simulink model "PARED_SIM_SFR"  (R2018a)
settings: Solver=ode45  StartTime=0.0  StopTime=30  RelTol=1e-6  AbsTol=1e-9  EnableMultiTasking=on
values from neighbouring files (symbols this model uses):
  d0 = 100    [CONTROL_SEGWAY.m]
  matAp = [-1/Tm_w 0 0 ; 1 0 0 ; 1000*xA 1000*va0 0]    [CONTROL_SEGWAY.m]
  matBp = [ Km_w/Tm_w 0 0; 0 -1 0; 0 0 0]    [CONTROL_SEGWAY.m]
  matCp = eye(3)    [CONTROL_SEGWAY.m]
  matDp = zeros(3,3)    [CONTROL_SEGWAY.m]
  param_pared = [Km_w Tm_w xA yA]    [CONTROL_SEGWAY.m]
  ts = 5e-3    (= 0.005)    [CONTROL_SEGWAY.m]
  va0 = 0.15    [CONTROL_SEGWAY.m]
undefined symbols (not defined in the file or in its folder): Kcd_pared
settings Model: Creator=zamora  LastModifiedBy=zamora
settings SolverCC: AutoScaleAbsTol=off
settings DataIOCC: LimitDataPoints=on  SaveFormat=Array  SignalLoggingSaveFormat=ModelDataLogs
settings OptimizationCC: ExpressionDepthLimit=2147483647  LifeSpan=inf
settings DebuggingCC: UnderspecifiedInitializationDetection=Classic  MergeDetectMultiDrivingBlocksExec=none  MultiTaskDSMMsg=warning  MultiTaskCondExecSysMsg=none  FcnCallInpInsideContextMsg=warning  StateNameClashWarn=warning  SFUnexpectedBacktrackingDiag=warning  SFNoUnconditionalDefaultTransitionDiag=warning  SFExecutionAtInitializationDiag=none
settings HardwareCC: ProdBitPerPointer=32  ProdBitPerSizeT=32  ProdBitPerPtrDiffT=32  ProdLargestAtomicFloat=None  ProdIntDivRoundTo=Undefined  ProdEndianess=Unspecified  ProdWordSize=32  ProdHWDeviceType=32-bit Generic
settings ModelReferenceCC: PropagateSignalLabelsOutOfModel=off
settings CodeAppCC: StateflowObjectComments=on
settings GRTTargetCC: TargetLangStandard=C89/C90 (ANSI)  GeneratePreprocessorConditionals=Disable all  CombineOutputUpdateFcns=off  GRTInterface=on
settings ConfigComp: CovMetricSettings=dw  CovHtmlReporting=on  CovSaveCumulativeToWorkspaceVar=on  CovSaveSingleToWorkspaceVar=on  CovExternalEMLEnable=off  CovSFcnEnable=off

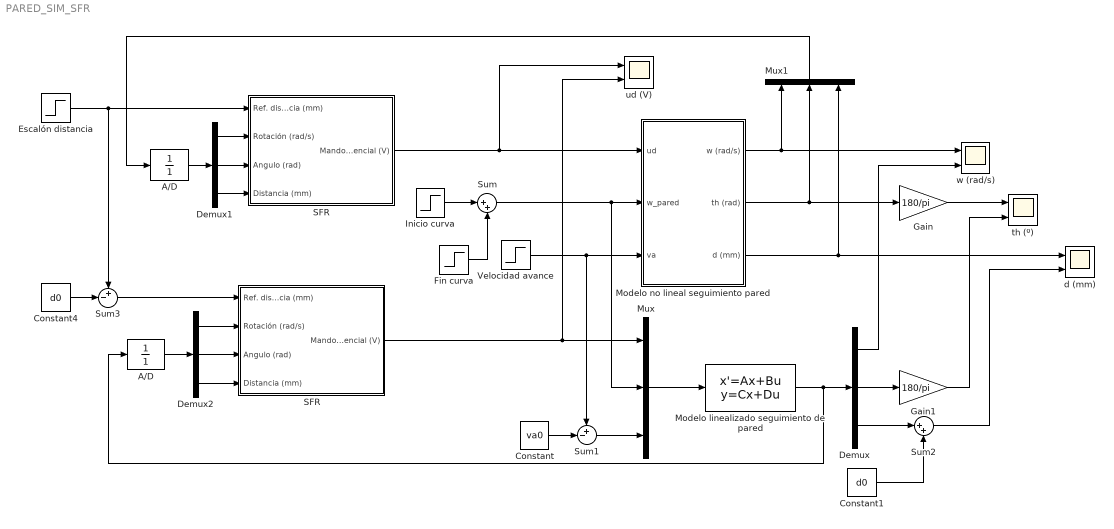
== system PARED_SIM_SFR ==
  A/D : DiscreteTransferFcn  Denominator=[1]  SampleTime=ts
  "A/D " : DiscreteTransferFcn  Denominator=[1]  SampleTime=ts
  Constant : Constant  Value=va0  SampleTime=0
  Constant1 : Constant  Value=d0  SampleTime=0
  Constant4 : Constant  Value=d0  SampleTime=ts
  Demux : Demux  Outputs=3
  Demux1 : Demux  Outputs=3
  Demux2 : Demux  Outputs=3
  Escalón distancia : Step  Time=5  Before=d0  After=d0*0.9  SampleTime=ts
  Fin curva : Step  Time=15  After=-va0/0.9  SampleTime=0
  Gain : Gain  Gain=180/pi
  Gain1 : Gain  Gain=180/pi
  Inicio curva : Step  Time=10  After=va0/0.9  SampleTime=0
  Modelo linealizado seguimiento de pared : StateSpace  A=matAp  B=matBp  C=matCp  D=matDp  InitialCondition=zeros(3,1)
  Modelo no lineal seguimiento pared : Subsystem
  Mux : Mux  Inputs=3
  Mux1 : Mux  Inputs=3
  SFR : Subsystem
  "SFR " : Subsystem
  Sum : Sum  Inputs=|++
  Sum1 : Sum  Inputs=+-|
  Sum2 : Sum  Inputs=|++
  Sum3 : Sum  Inputs=+-|
  Velocidad avance : Step  Time=20  Before=va0  After=va0*0.75  SampleTime=0
  d (mm) : Scope  NumInputPorts=2
  th (º) : Scope  NumInputPorts=2
  ud (V) : Scope  NumInputPorts=2
  w (rad/s) : Scope  NumInputPorts=2
  wires:
  Inicio curva/1 -> Sum/1
  Fin curva/1 -> Sum/2
  Mux/1 -> Modelo linealizado seguimiento de pared/1
  Velocidad avance/1 -> Modelo no lineal seguimiento pared/3(va), Sum1/1
  Constant/1 -> Sum1/2
  SFR/1(Mando diferencial (V)) -> ud (V)/1, Modelo no lineal seguimiento pared/1(ud)
  Modelo linealizado seguimiento de pared/1 -> "A/D "/1, Demux/1
  Modelo no lineal seguimiento pared/1(w (rad/s)) -> Mux1/1, w (rad/s)/1
  Demux/1 -> w (rad/s)/2
  Modelo no lineal seguimiento pared/2(th (rad)) -> Mux1/2, Gain/1
  Gain/1 -> th (º)/1
  Demux/2 -> Gain1/1
  Gain1/1 -> th (º)/2
  Demux/3 -> Sum2/1
  Constant1/1 -> Sum2/2
  Sum2/1 -> d (mm)/2
  Modelo no lineal seguimiento pared/3(d (mm)) -> Mux1/3, d (mm)/1
  "SFR "/1(Mando diferencial (V)) -> ud (V)/2, Mux/1
  Sum3/1 -> "SFR "/1(Ref. distancia (mm))
  Constant4/1 -> Sum3/2
  Escalón distancia/1 -> SFR/1(Ref. distancia (mm)), Sum3/1
  Demux1/1 -> SFR/2(Rotación (rad/s))
  Demux1/2 -> SFR/3(Angulo (rad))
  Demux1/3 -> SFR/4(Distancia (mm))
  Demux2/1 -> "SFR "/2(Rotación (rad/s))
  Demux2/2 -> "SFR "/3(Angulo (rad))
  Demux2/3 -> "SFR "/4(Distancia (mm))
  Mux1/1 -> A/D/1
  A/D/1 -> Demux1/1
  "A/D "/1 -> Demux2/1
  Sum1/1 -> Mux/3
  Sum/1 -> Mux/2, Modelo no lineal seguimiento pared/2(w_pared)

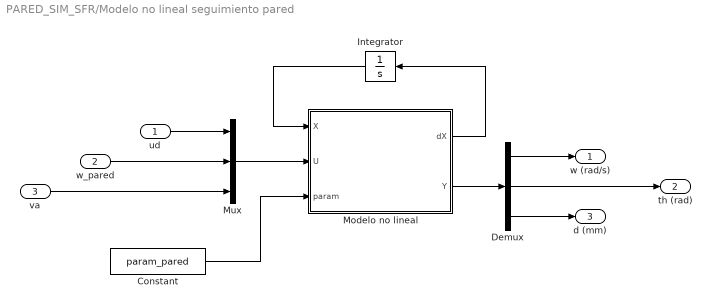
== system PARED_SIM_SFR/Modelo no lineal seguimiento pared ==
  ud : Inport
  w_pared : Inport  Port=2
  va : Inport  Port=3
  Constant : Constant  Value=param_pared  SampleTime=0
  Demux : Demux  Outputs=3
  Integrator : Integrator  InitialCondition=[0 0 d0]'
  Modelo no lineal : MATLAB Function  TreatAsAtomicUnit=on
  Mux : Mux  Inputs=3
  w (rad/s) : Outport
  th (rad) : Outport  Port=2
  d (mm) : Outport  Port=3
  wires:
  Constant/1 -> Modelo no lineal/3(param)
  Demux/1 -> w (rad/s)/1
  Demux/2 -> th (rad)/1
  Mux/1 -> Modelo no lineal/2(U)
  Integrator/1 -> Modelo no lineal/1(X)
  Modelo no lineal/1(dX) -> Integrator/1
  Modelo no lineal/2(Y) -> Demux/1
  ud/1 -> Mux/1
  Demux/3 -> d (mm)/1
  va/1 -> Mux/3
  w_pared/1 -> Mux/2

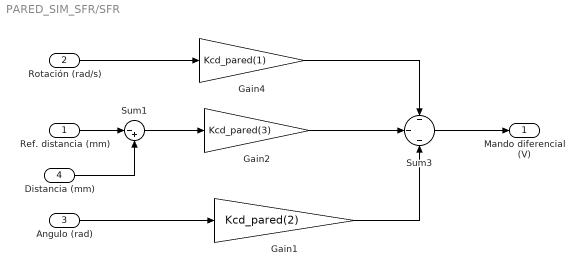
== system PARED_SIM_SFR/SFR ==
  Ref. distancia (mm) : Inport
  Rotación (rad/s) : Inport  Port=2
  Angulo (rad) : Inport  Port=3
  Distancia (mm) : Inport  Port=4
  Gain1 : Gain  Gain=Kcd_pared(2)
  Gain2 : Gain  Gain=Kcd_pared(3)
  Gain4 : Gain  Gain=Kcd_pared(1)
  Sum1 : Sum  Inputs=|-+
  Sum3 : Sum  Inputs=-|-|-
  Mando diferencial (V) : Outport
  wires:
  Sum1/1 -> Gain2/1
  Gain1/1 -> Sum3/3
  Gain4/1 -> Sum3/1
  Rotación (rad/s)/1 -> Gain4/1
  Angulo (rad)/1 -> Gain1/1
  Sum3/1 -> Mando diferencial (V)/1
  Ref. distancia (mm)/1 -> Sum1/1
  Gain2/1 -> Sum3/2
  Distancia (mm)/1 -> Sum1/2

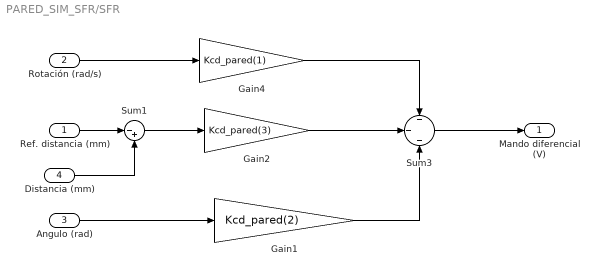
== system PARED_SIM_SFR/SFR  ==
  Ref. distancia (mm) : Inport
  Rotación (rad/s) : Inport  Port=2
  Angulo (rad) : Inport  Port=3
  Distancia (mm) : Inport  Port=4
  Gain1 : Gain  Gain=Kcd_pared(2)
  Gain2 : Gain  Gain=Kcd_pared(3)
  Gain4 : Gain  Gain=Kcd_pared(1)
  Sum1 : Sum  Inputs=|-+
  Sum3 : Sum  Inputs=-|-|-
  Mando diferencial (V) : Outport
  wires:
  Distancia (mm)/1 -> Sum1/2
  Gain2/1 -> Sum3/2
  Ref. distancia (mm)/1 -> Sum1/1
  Angulo (rad)/1 -> Gain1/1
  Rotación (rad/s)/1 -> Gain4/1
  Gain4/1 -> Sum3/1
  Gain1/1 -> Sum3/3
  Sum1/1 -> Gain2/1
  Sum3/1 -> Mando diferencial (V)/1

== matlab function PARED_SIM_SFR/Modelo no lineal seguimiento pared/Modelo no lineal ==
  data: X input; dX output; U input; param input; Y output
function [dX,Y] = segway_pared(X,U,param)

%% Parametros
% Ganancia estática giro (rad/s/V)
Km_w=param(1);
% Constante de tiempo giro (s)
Tm_w=param(2);
% Abcisa punto A (m)
xA=param(3);
% Ordenada punto A (m)
yA=param(4);

%% Entradas
% Tension diferencial (V)
ud=U(1);
% Velocidad angular de la pared (rad/s)
w_pared=U(2);
% Velocidad de avance (m/s)
va=U(3);

%% Variables de estado
% Velocidad angular del vehículo  (m/s)
w=X(1);
% Angulo del vehículo con respecto a la pared (rad)
th=X(2);
% Distancia a la pared (mm)
d=X(3);

%% Ecuaciones de estado
dw = -1/Tm_w*w + Km_w/Tm_w*ud;
dth = w - w_pared;
dd = 1000*(va-w*yA)*sin(th) + 1000*w*xA*cos(th);
% Derivada del vector de estado
dX=[dw dth dd]';

%% Ecuaciones de salida
Y = X;
